simulink model "SimulacaoMotorCCr2016a"  (R2018a)
settings: Solver=FixedStepAuto  StartTime=0.0  StopTime=0.23  RelTol=1e-4
values from neighbouring files (symbols this model uses):
  B = 0.0006    [ParameterEstimation.m]
  J = 0.00050804    [ParameterEstimation.m]
  K = 0.087    [ParameterEstimation.m]
  La = 0.000150    (= 0.00015)    [ParameterEstimation.m]
  Ra = 0.1501    [ParameterEstimation.m]
  Ts = 1e-4    (= 0.0001)    [ParameterEstimation.m]
Description:
  | Sistema de injeção completo.
settings Model: ExtModeAutoUpdateStatusClock=off  Creator=vtchkalo  LastModifiedBy=joaovitor
settings SolverCC: MaxConsecutiveZCs=100000  ZeroCrossAlgorithm=Adaptive
settings DataIOCC: LimitDataPoints=on  SaveFormat=Array  SaveState=on  SignalLogging=off  DSMLogging=off  OutputOption=SpecifiedOutputTimes  OutputTimes=SDO_OutputTimes  ReturnWorkspaceOutputsName=SDOSimTest_Log
settings OptimizationCC: BlockReduction=off  BooleanDataType=off  LifeSpan=inf
settings DebuggingCC: SaveWithParameterizedLinksMsg=none  UnderspecifiedInitializationDetection=Classic  MergeDetectMultiDrivingBlocksExec=none  SignalResolutionControl=TryResolveAllWithWarning  MultiTaskDSMMsg=warning  MultiTaskCondExecSysMsg=none  StateNameClashWarn=warning  SFUnexpectedBacktrackingDiag=warning  SFNoUnconditionalDefaultTransitionDiag=warning  SFExecutionAtInitializationDiag=none
settings HardwareCC: ProdBitPerPointer=32  ProdBitPerSizeT=32  ProdBitPerPtrDiffT=32  ProdLargestAtomicFloat=None  ProdIntDivRoundTo=Undefined  ProdEndianess=Unspecified  ProdWordSize=32  ProdHWDeviceType=32-bit Generic  TargetUnknown=on
settings ModelReferenceCC: PropagateSignalLabelsOutOfModel=off
settings CodeAppCC: StateflowObjectComments=on
settings GRTTargetCC: TargetLangStandard=C89/C90 (ANSI)
settings ConfigComp: CovMetricSettings=dw  CovHtmlReporting=on  CovSaveCumulativeToWorkspaceVar=on  CovSaveSingleToWorkspaceVar=on  CovExternalEMLEnable=off
settings SimscapeCC: SimscapeNormalizeSystem=off

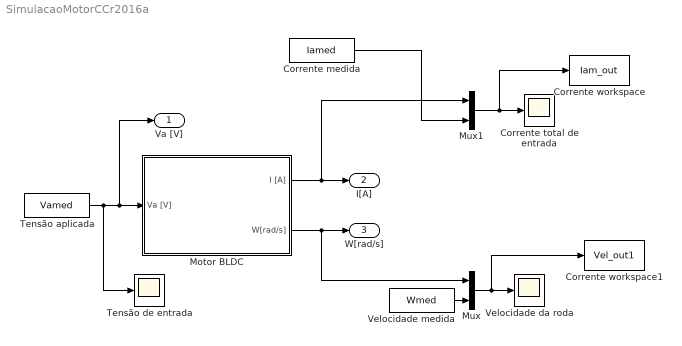
== system SimulacaoMotorCCr2016a ==
  Corrente medida : FromWorkspace  VariableName=Iamed  SampleTime=Ts
  Corrente total de entrada : Scope
  Corrente workspace : ToWorkspace  VariableName=Iam_out  SaveFormat=Timeseries  SampleTime=-1
  Corrente workspace1 : ToWorkspace  VariableName=Vel_out1  SaveFormat=Timeseries  SampleTime=-1
  Motor BLDC : Subsystem
  Mux : Mux  Inputs=2
  Mux1 : Mux  Inputs=2
  Tensão aplicada : FromWorkspace  VariableName=Vamed  SampleTime=Ts
  Tensão de entrada : Scope
  Velocidade da roda : Scope
  Velocidade medida : FromWorkspace  VariableName=Wmed  SampleTime=Ts
  Va [V] : Outport
  I[A] : Outport  Port=2
  W[rad/s] : Outport  Port=3
  wires:
  Tensão aplicada/1 -> Motor BLDC/1(Va [V]), Va [V]/1, Tensão de entrada/1
  Velocidade medida/1 -> Mux/2
  Mux/1 -> Corrente workspace1/1, Velocidade da roda/1
  Mux1/1 -> Corrente workspace/1, Corrente total de entrada/1
  Corrente medida/1 -> Mux1/2
  Motor BLDC/1(I [A]) -> Mux1/1, I[A]/1
  Motor BLDC/2(W[rad/s]) -> Mux/1, W[rad/s]/1

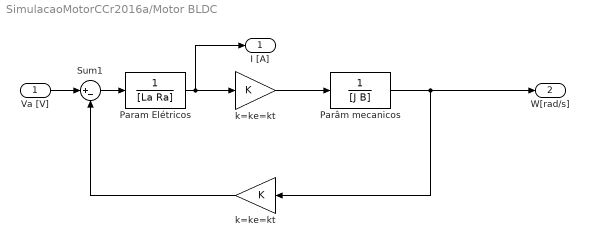
== system SimulacaoMotorCCr2016a/Motor BLDC ==
  Va [V] : Inport
  Param Elétricos : TransferFcn  Denominator=[La Ra]
  Parâm mecanicos : TransferFcn  Denominator=[J B]
  Sum1 : Sum  Inputs=|+-
  k=ke=kt : Gain  Gain=K
  "k=ke=kt " : Gain  Gain=K
  I [A] : Outport
  W[rad/s] : Outport  Port=2
  wires:
  Sum1/1 -> Param Elétricos/1
  Va [V]/1 -> Sum1/1
  k=ke=kt/1 -> Sum1/2
  "k=ke=kt "/1 -> Parâm mecanicos/1
  Param Elétricos/1 -> I [A]/1, "k=ke=kt "/1
  Parâm mecanicos/1 -> W[rad/s]/1, k=ke=kt/1
